simulink model "SDHDummy_IK"  (R2023b)
settings: Solver=VariableStepAuto  StartTime=0.0  StopTime=15  RelTol=1e-3
values from neighbouring files (symbols this model uses):
  m = 0.1062    [Test_New_ROBOT_dynamics.m]
  M3 = [ ... (first row only)    [ForwardPOE_Test.m]    (also in ForwardPOE_Test_2.m; Make_Mlist_2.m = M_cell{3}; Make_Slist.m = [1.00000, 0.00000, 0.00000, 0.00000; 0.00000, 0.00000, 1.000; Mlist.m = eye(4))
  T = [1 0 0 0 ... (first row only)    [DH_to_Mlist.m]    (also in ForwardKinematics.m = [T3, Gtheta * se3mat(1:3, 4) / theta; 0, 0, 0, 1]; InverseDynamics.m = [R, p; 0 0 0 1]; SDHDummy_Circle.m = transl(P(i,:)) * rpy2tr(0, 0, pi, 'xyz'); SDHDummy_Heart.m = transl(P(i,:)) * rpy2tr(0, 0, pi, 'xyz'))
  T0 = [ ... (first row only)    [SDH_Main.m]
undefined symbols (not defined in the file or in its folder): Dummy, smiData, X, Y, Z
libraries: sm_lib x594, fl_lib x22, nesl_utility x13, simulink_extras x2, robotcorelib x1
(part 11 of 11)

== system SDHDummy_IK/Subsystem/J6_STEP_1_RIGID/x35_20Motor_Assembly_1_STEP_1_RIGID/x35Motor_Driver_2_STEP_1_RIGID ==
  Dummy_0020_STEP_1_RIGID : Subsystem
  Dummy_0021_STEP_1_RIGID : Subsystem
  ReferenceFrame : sm_lib/Frames and Transforms/Reference Frame
  Transform : sm_lib/Frames and Transforms/Rigid Transform  TranslationMethod=Cartesian  TranslationStandardOffset=0  TranslationStandardOffsetUnits=m  TranslationStandardAxis=+Z  TranslationCartesianOffset=smiData.RigidTransform(111).translation  TranslationCartesianOffsetUnits=mm  TranslationROffset=0  TranslationROffsetUnits=m  TranslationZOffset=0  TranslationZOffsetUnits=m  TranslationThetaOffset=0  TranslationThetaOffsetUnits=deg  RotationMethod=ArbitraryAxis  RotationAngleUnits=rad  RotationStandardAxis=+Z  RotationAngle=smiData.RigidTransform(111).angle  RotationArbitraryAxis=smiData.RigidTransform(111).axis  FollAlignAxisA=+X  BaseAlignAxisA=+Y  FollAlignAxisB=+Y  BaseAlignAxisB=+Z  RotationSequenceAxes=FollowerAxes  RotationSequence=XYX  RotationSequenceAngles=[0 0 0]  RotationSequenceAnglesUnits=deg  RotationMatrix=[1 0 0; 0 1 0; 0 0 1]  Quaternion=[1 0 0 0]
  Transform1 : sm_lib/Frames and Transforms/Rigid Transform  TranslationMethod=Cartesian  TranslationStandardOffset=0  TranslationStandardOffsetUnits=m  TranslationStandardAxis=+Z  TranslationCartesianOffset=smiData.RigidTransform(112).translation  TranslationCartesianOffsetUnits=mm  TranslationROffset=0  TranslationROffsetUnits=m  TranslationZOffset=0  TranslationZOffsetUnits=m  TranslationThetaOffset=0  TranslationThetaOffsetUnits=deg  RotationMethod=ArbitraryAxis  RotationAngleUnits=rad  RotationStandardAxis=+Z  RotationAngle=smiData.RigidTransform(112).angle  RotationArbitraryAxis=smiData.RigidTransform(112).axis  FollAlignAxisA=+X  BaseAlignAxisA=+Y  FollAlignAxisB=+Y  BaseAlignAxisB=+Z  RotationSequenceAxes=FollowerAxes  RotationSequence=XYX  RotationSequenceAngles=[0 0 0]  RotationSequenceAnglesUnits=deg  RotationMatrix=[1 0 0; 0 1 0; 0 0 1]  Quaternion=[1 0 0 0]
  Transform2 : sm_lib/Frames and Transforms/Rigid Transform  TranslationMethod=Cartesian  TranslationStandardOffset=0  TranslationStandardOffsetUnits=m  TranslationStandardAxis=+Z  TranslationCartesianOffset=smiData.RigidTransform(113).translation  TranslationCartesianOffsetUnits=mm  TranslationROffset=0  TranslationROffsetUnits=m  TranslationZOffset=0  TranslationZOffsetUnits=m  TranslationThetaOffset=0  TranslationThetaOffsetUnits=deg  RotationMethod=ArbitraryAxis  RotationAngleUnits=rad  RotationStandardAxis=+Z  RotationAngle=smiData.RigidTransform(113).angle  RotationArbitraryAxis=smiData.RigidTransform(113).axis  FollAlignAxisA=+X  BaseAlignAxisA=+Y  FollAlignAxisB=+Y  BaseAlignAxisB=+Z  RotationSequenceAxes=FollowerAxes  RotationSequence=XYX  RotationSequenceAngles=[0 0 0]  RotationSequenceAnglesUnits=deg  RotationMatrix=[1 0 0; 0 1 0; 0 0 1]  Quaternion=[1 0 0 0]
  F : PMIOPort  Side=Left
  connections:
  Dummy_0020_STEP_1_RIGID/LConn1 -- Transform/RConn1
  Dummy_0021_STEP_1_RIGID/LConn1 -- Transform1/RConn1
  ReferenceFrame/RConn1 -- Transform/LConn1 -- Transform1/LConn1 -- Transform2/RConn1
  Transform2/LConn1 -- F/RConn1

== system SDHDummy_IK/Subsystem/J6_STEP_1_RIGID/x35_20Motor_Assembly_1_STEP_1_RIGID/x35_20_STEP_1_RIGID ==
  ReferenceFrame : sm_lib/Frames and Transforms/Reference Frame
  Solid : sm_lib/Body Elements/File Solid  ExtGeomFileName=35-20步进电机.STEP_默认_sldprt.STEP  UnitType=FromFile  ExtGeomFileUnits=m  StepReaderType=HEX  ExportConvexHullGeometry=off  InertiaType=Custom  Mass=smiData.Solid(31).mass  MassUnits=kg  CenterOfMass=smiData.Solid(31).CoM  CenterOfMassUnits=mm  MomentsOfInertia=smiData.Solid(31).MoI  MomentsOfInertiaUnits=kg*mm^2  ProductsOfInertia=smiData.Solid(31).PoI  ProductsOfInertiaUnits=kg*mm^2  BasedOnType=DensityFromFile  Density=1000  DensityUnits=kg/m^3  DoExposeReferenceFrame=on  SerializedFrames=<Frames/>  GraphicType=FromGeometry  MarkerShape=Sphere  MarkerSize=10  GraphicVisPropType=SimpleVisualProperties  GraphicDiffuseColor=smiData.Solid(31).color  GraphicSpecularColor=[0.5 0.5 0.5 1.0]  GraphicAmbientColor=[0.15 0.15 0.15 1.0]  GraphicEmissiveColor=[0.0 0.0 0.0 1.0]  GraphicShininess=75  GraphicOpacity=smiData.Solid(31).opacity
  F : PMIOPort  Side=Left
  connections:
  ReferenceFrame/RConn1 -- Solid/RConn1 -- F/RConn1

== system SDHDummy_IK/Subsystem/J4_STEP_1_RIGID/x35_28Motor_Assembly_STEP_1_RIGID/x35Motor_Driver_STEP_1_RIGID/Dummy_0020_STEP_1_RIGID ==
  ReferenceFrame : sm_lib/Frames and Transforms/Reference Frame
  Solid : sm_lib/Body Elements/File Solid  ExtGeomFileName=Dummy-0020.STEP_默认_sldprt.STEP  UnitType=FromFile  ExtGeomFileUnits=m  StepReaderType=HEX  ExportConvexHullGeometry=off  InertiaType=Custom  Mass=smiData.Solid(23).mass  MassUnits=kg  CenterOfMass=smiData.Solid(23).CoM  CenterOfMassUnits=mm  MomentsOfInertia=smiData.Solid(23).MoI  MomentsOfInertiaUnits=kg*mm^2  ProductsOfInertia=smiData.Solid(23).PoI  ProductsOfInertiaUnits=kg*mm^2  BasedOnType=DensityFromFile  Density=1000  DensityUnits=kg/m^3  DoExposeReferenceFrame=on  SerializedFrames=<Frames/>  GraphicType=FromGeometry  MarkerShape=Sphere  MarkerSize=10  GraphicVisPropType=SimpleVisualProperties  GraphicDiffuseColor=smiData.Solid(23).color  GraphicSpecularColor=[0.5 0.5 0.5 1.0]  GraphicAmbientColor=[0.15 0.15 0.15 1.0]  GraphicEmissiveColor=[0.0 0.0 0.0 1.0]  GraphicShininess=75  GraphicOpacity=smiData.Solid(23).opacity
  F : PMIOPort  Side=Left
  connections:
  ReferenceFrame/RConn1 -- Solid/RConn1 -- F/RConn1

== system SDHDummy_IK/Subsystem/J4_STEP_1_RIGID/x35_28Motor_Assembly_STEP_1_RIGID/x35Motor_Driver_STEP_1_RIGID/Dummy_0021_STEP_1_RIGID ==
  ReferenceFrame : sm_lib/Frames and Transforms/Reference Frame
  Solid : sm_lib/Body Elements/File Solid  ExtGeomFileName=Dummy-0021.STEP_默认_sldprt.STEP  UnitType=FromFile  ExtGeomFileUnits=m  StepReaderType=HEX  ExportConvexHullGeometry=off  InertiaType=Custom  Mass=smiData.Solid(24).mass  MassUnits=kg  CenterOfMass=smiData.Solid(24).CoM  CenterOfMassUnits=mm  MomentsOfInertia=smiData.Solid(24).MoI  MomentsOfInertiaUnits=kg*mm^2  ProductsOfInertia=smiData.Solid(24).PoI  ProductsOfInertiaUnits=kg*mm^2  BasedOnType=DensityFromFile  Density=1000  DensityUnits=kg/m^3  DoExposeReferenceFrame=on  SerializedFrames=<Frames/>  GraphicType=FromGeometry  MarkerShape=Sphere  MarkerSize=10  GraphicVisPropType=SimpleVisualProperties  GraphicDiffuseColor=smiData.Solid(24).color  GraphicSpecularColor=[0.5 0.5 0.5 1.0]  GraphicAmbientColor=[0.15 0.15 0.15 1.0]  GraphicEmissiveColor=[0.0 0.0 0.0 1.0]  GraphicShininess=75  GraphicOpacity=smiData.Solid(24).opacity
  F : PMIOPort  Side=Left
  connections:
  ReferenceFrame/RConn1 -- Solid/RConn1 -- F/RConn1

== system SDHDummy_IK/Subsystem/J5_STEP_1_RIGID/x35_20Motor_Assembly_STEP_1_RIGID/x35Motor_Driver_1_STEP_1_RIGID/Dummy_0020_STEP_1_RIGID ==
  ReferenceFrame : sm_lib/Frames and Transforms/Reference Frame
  Solid : sm_lib/Body Elements/File Solid  ExtGeomFileName=Dummy-0020.STEP_默认_sldprt.STEP  UnitType=FromFile  ExtGeomFileUnits=m  StepReaderType=HEX  ExportConvexHullGeometry=off  InertiaType=Custom  Mass=smiData.Solid(23).mass  MassUnits=kg  CenterOfMass=smiData.Solid(23).CoM  CenterOfMassUnits=mm  MomentsOfInertia=smiData.Solid(23).MoI  MomentsOfInertiaUnits=kg*mm^2  ProductsOfInertia=smiData.Solid(23).PoI  ProductsOfInertiaUnits=kg*mm^2  BasedOnType=DensityFromFile  Density=1000  DensityUnits=kg/m^3  DoExposeReferenceFrame=on  SerializedFrames=<Frames/>  GraphicType=FromGeometry  MarkerShape=Sphere  MarkerSize=10  GraphicVisPropType=SimpleVisualProperties  GraphicDiffuseColor=smiData.Solid(23).color  GraphicSpecularColor=[0.5 0.5 0.5 1.0]  GraphicAmbientColor=[0.15 0.15 0.15 1.0]  GraphicEmissiveColor=[0.0 0.0 0.0 1.0]  GraphicShininess=75  GraphicOpacity=smiData.Solid(23).opacity
  F : PMIOPort  Side=Left
  connections:
  ReferenceFrame/RConn1 -- Solid/RConn1 -- F/RConn1

== system SDHDummy_IK/Subsystem/J5_STEP_1_RIGID/x35_20Motor_Assembly_STEP_1_RIGID/x35Motor_Driver_1_STEP_1_RIGID/Dummy_0021_STEP_1_RIGID ==
  ReferenceFrame : sm_lib/Frames and Transforms/Reference Frame
  Solid : sm_lib/Body Elements/File Solid  ExtGeomFileName=Dummy-0021.STEP_默认_sldprt.STEP  UnitType=FromFile  ExtGeomFileUnits=m  StepReaderType=HEX  ExportConvexHullGeometry=off  InertiaType=Custom  Mass=smiData.Solid(24).mass  MassUnits=kg  CenterOfMass=smiData.Solid(24).CoM  CenterOfMassUnits=mm  MomentsOfInertia=smiData.Solid(24).MoI  MomentsOfInertiaUnits=kg*mm^2  ProductsOfInertia=smiData.Solid(24).PoI  ProductsOfInertiaUnits=kg*mm^2  BasedOnType=DensityFromFile  Density=1000  DensityUnits=kg/m^3  DoExposeReferenceFrame=on  SerializedFrames=<Frames/>  GraphicType=FromGeometry  MarkerShape=Sphere  MarkerSize=10  GraphicVisPropType=SimpleVisualProperties  GraphicDiffuseColor=smiData.Solid(24).color  GraphicSpecularColor=[0.5 0.5 0.5 1.0]  GraphicAmbientColor=[0.15 0.15 0.15 1.0]  GraphicEmissiveColor=[0.0 0.0 0.0 1.0]  GraphicShininess=75  GraphicOpacity=smiData.Solid(24).opacity
  F : PMIOPort  Side=Left
  connections:
  ReferenceFrame/RConn1 -- Solid/RConn1 -- F/RConn1

== system SDHDummy_IK/Subsystem/J6_STEP_1_RIGID/x35_20Motor_Assembly_1_STEP_1_RIGID/x35Motor_Driver_2_STEP_1_RIGID/Dummy_0020_STEP_1_RIGID ==
  ReferenceFrame : sm_lib/Frames and Transforms/Reference Frame
  Solid : sm_lib/Body Elements/File Solid  ExtGeomFileName=Dummy-0020.STEP_默认_sldprt.STEP  UnitType=FromFile  ExtGeomFileUnits=m  StepReaderType=HEX  ExportConvexHullGeometry=off  InertiaType=Custom  Mass=smiData.Solid(23).mass  MassUnits=kg  CenterOfMass=smiData.Solid(23).CoM  CenterOfMassUnits=mm  MomentsOfInertia=smiData.Solid(23).MoI  MomentsOfInertiaUnits=kg*mm^2  ProductsOfInertia=smiData.Solid(23).PoI  ProductsOfInertiaUnits=kg*mm^2  BasedOnType=DensityFromFile  Density=1000  DensityUnits=kg/m^3  DoExposeReferenceFrame=on  SerializedFrames=<Frames/>  GraphicType=FromGeometry  MarkerShape=Sphere  MarkerSize=10  GraphicVisPropType=SimpleVisualProperties  GraphicDiffuseColor=smiData.Solid(23).color  GraphicSpecularColor=[0.5 0.5 0.5 1.0]  GraphicAmbientColor=[0.15 0.15 0.15 1.0]  GraphicEmissiveColor=[0.0 0.0 0.0 1.0]  GraphicShininess=75  GraphicOpacity=smiData.Solid(23).opacity
  F : PMIOPort  Side=Left
  connections:
  ReferenceFrame/RConn1 -- Solid/RConn1 -- F/RConn1

== system SDHDummy_IK/Subsystem/J6_STEP_1_RIGID/x35_20Motor_Assembly_1_STEP_1_RIGID/x35Motor_Driver_2_STEP_1_RIGID/Dummy_0021_STEP_1_RIGID ==
  ReferenceFrame : sm_lib/Frames and Transforms/Reference Frame
  Solid : sm_lib/Body Elements/File Solid  ExtGeomFileName=Dummy-0021.STEP_默认_sldprt.STEP  UnitType=FromFile  ExtGeomFileUnits=m  StepReaderType=HEX  ExportConvexHullGeometry=off  InertiaType=Custom  Mass=smiData.Solid(24).mass  MassUnits=kg  CenterOfMass=smiData.Solid(24).CoM  CenterOfMassUnits=mm  MomentsOfInertia=smiData.Solid(24).MoI  MomentsOfInertiaUnits=kg*mm^2  ProductsOfInertia=smiData.Solid(24).PoI  ProductsOfInertiaUnits=kg*mm^2  BasedOnType=DensityFromFile  Density=1000  DensityUnits=kg/m^3  DoExposeReferenceFrame=on  SerializedFrames=<Frames/>  GraphicType=FromGeometry  MarkerShape=Sphere  MarkerSize=10  GraphicVisPropType=SimpleVisualProperties  GraphicDiffuseColor=smiData.Solid(24).color  GraphicSpecularColor=[0.5 0.5 0.5 1.0]  GraphicAmbientColor=[0.15 0.15 0.15 1.0]  GraphicEmissiveColor=[0.0 0.0 0.0 1.0]  GraphicShininess=75  GraphicOpacity=smiData.Solid(24).opacity
  F : PMIOPort  Side=Left
  connections:
  ReferenceFrame/RConn1 -- Solid/RConn1 -- F/RConn1

== matlab function SDHDummy_IK/MATLAB Function ==
  data: all_solutions input; optimal_joint output; current_joint input
function optimal_joint = ur5_select_optimal_simple(all_solutions, current_joint)
%#codegen
%UR5_SELECT_OPTIMAL_SIMPLE 从8组逆解中选择最优解（简化版）
%
%   输入:
%       all_solutions - 8x6 矩阵，8组可能的关节角解 (rad)
%       current_joint - 1x6 向量，当前关节角度 (rad)
%
%   输出:
%       optimal_joint - 1x6 向量，最优的关节角解 (rad)
%
%   选择准则:  选择与当前关节角度变化最小的有效解

    %% ================== 初始化 ==================
    NUM_SOLUTIONS = 8;
    NUM_JOINTS = 6;
    
    optimal_joint = zeros(1, NUM_JOINTS);
    min_distance = 1e10;
    best_idx = 0;

    %% ================== 遍历所有解 ==================
    for sol_idx = 1:NUM_SOLUTIONS
        
        % 检查是否为有效解（无NaN/Inf）
        is_valid = true;
        for j = 1:NUM_JOINTS
            if isnan(all_solutions(sol_idx, j)) || isinf(all_solutions(sol_idx, j))
                is_valid = false;
            end
        end
        
        if ~is_valid
            continue;
        end
        
        % 计算与当前关节角度的距离
        distance = 0;
        for j = 1:NUM_JOINTS
            % 角度差归一化
            diff = all_solutions(sol_idx, j) - current_joint(j);
            
            while diff > pi
                diff = diff - 2*pi;
            end
            while diff < -pi
                diff = diff + 2*pi;
            end
            
            distance = distance + diff^2;
        end
        distance = sqrt(distance);
        
        % 更新最优解
        if distance < min_distance
            min_distance = distance;
            best_idx = sol_idx;
        end
    end

    %% ================== 输出结果 ==================
    if best_idx > 0
        for j = 1:NUM_JOINTS
            ang = all_solutions(best_idx, j);
            while ang > pi
                ang = ang - 2*pi;
            end
            while ang < -pi
                ang = ang + 2*pi;
            end
            optimal_joint(j) = ang;
        end
    else
        % 无有效解，返回当前角度
        for j = 1:NUM_JOINTS
            optimal_joint(j) = current_joint(j);
        end
    end

end

== matlab function SDHDummy_IK/MATLAB Function2 ==
  data: q input; T_06 output
function T_06 = FKfcn(q)
% 输入 q: 关节角度向量 [theta1, theta2, theta3, theta4, theta5, theta6] (弧度)
% 输出 T_06: 末端执行器的 4x4 齐次变换矩阵

    % DH 参数定义 (根据你提供的数据)
    % theta(变量), d, a, alpha
    % 注意：q(i) 将替代 DH 表中的 theta 值
    
    %         d         a        alpha
    DH_params = [
        0.1245    0.035    -pi/2;  % Link 1
        0         0.146     0;     % Link 2
        0         0.052    -pi/2;  % Link 3
        0.117     0         pi/2;  % Link 4
        0         0        -pi/2;  % Link 5
        0.0775    0         0      % Link 6
    ];

    % 初始化变换矩阵为单位矩阵
    T_06 = eye(4);

    % 循环计算每一个连杆的变换矩阵并连乘
    % T_total = T_01 * T_12 * T_23 * T_34 * T_45 * T_56
    for i = 1:6
        theta = q(i);           % 当前关节角
        d     = DH_params(i, 1);
        a     = DH_params(i, 2);
        alpha = DH_params(i, 3);
        
        % 预计算三角函数以提高效率
        ct = cos(theta);
        st = sin(theta);
        ca = cos(alpha);
        sa = sin(alpha);
        
        % 标准 DH (Standard DH) 变换矩阵公式
        % T(i-1 -> i) = Rot_z(theta) * Trans_z(d) * Trans_x(a) * Rot_x(alpha)
        Ti = [
            ct,   -st*ca,   st*sa,   a*ct;
            st,    ct*ca,  -ct*sa,   a*st;
             0,       sa,      ca,      d;
             0,        0,       0,      1
        ];
        
        % 矩阵链乘
        T_06 = T_06 * Ti;
    end
end

== matlab function SDHDummy_IK/MATLAB Function3 ==
  data: q input; T_06 output
function T_06 = FKfcn(q)
% 输入 q: 关节角度向量 [theta1, theta2, theta3, theta4, theta5, theta6] (弧度)
% 输出 T_06: 末端执行器的 4x4 齐次变换矩阵

    % DH 参数定义 (根据你提供的数据)
    % theta(变量), d, a, alpha
    % 注意：q(i) 将替代 DH 表中的 theta 值
    
    %         d         a        alpha
    DH_params = [
        0.1245    0.035    -pi/2;  % Link 1
        0         0.146     0;     % Link 2
        0         0.052    -pi/2;  % Link 3
        0.117     0         pi/2;  % Link 4
        0         0        -pi/2;  % Link 5
        0.0775    0         0      % Link 6
    ];

    % 初始化变换矩阵为单位矩阵
    T_06 = eye(4);

    % 循环计算每一个连杆的变换矩阵并连乘
    % T_total = T_01 * T_12 * T_23 * T_34 * T_45 * T_56
    for i = 1:6
        theta = q(i);           % 当前关节角
        d     = DH_params(i, 1);
        a     = DH_params(i, 2);
        alpha = DH_params(i, 3);
        
        % 预计算三角函数以提高效率
        ct = cos(theta);
        st = sin(theta);
        ca = cos(alpha);
        sa = sin(alpha);
        
        % 标准 DH (Standard DH) 变换矩阵公式
        % T(i-1 -> i) = Rot_z(theta) * Trans_z(d) * Trans_x(a) * Rot_x(alpha)
        Ti = [
            ct,   -st*ca,   st*sa,   a*ct;
            st,    ct*ca,  -ct*sa,   a*st;
             0,       sa,      ca,      d;
             0,        0,       0,      1
        ];
        
        % 矩阵链乘
        T_06 = T_06 * Ti;
    end
end

== matlab function SDHDummy_IK/MATLAB Function1 ==
  data: T input; joint_angles output; DH_params input
function joint_angles = spherical_wrist_inverse_kinematics(T, DH_params)
%#codegen
%SPHERICAL_WRIST_INVERSE_KINEMATICS 球形腕机械臂逆运动学解析解（Simulink兼容）
%
%   输入:  
%       T         - 4x4 齐次变换矩阵，表示末端执行器位姿
%       DH_params - 6x4 DH参数矩阵 [a, d, alpha, theta_offset]
%                   或 1x6 向量 [a1, a2, a3, d1, d4, d6] (简化输入)
%
%   输出:
%       joint_angles - 8x6 矩阵，每行为一组可能的关节角解 [θ1,θ2,θ3,θ4,θ5,θ6] (rad)
%
%   适用条件: 
%       腕部三轴相交（Pieper准则）的6轴机械臂
%       
%   解的结构 (8组解):
%       θ1: 2个解 (左臂/右臂)
%       θ3: 2个解 (肘上/肘下)  
%       θ5: 2个解 (腕正/腕反)

    %% ================== 提取DH参数 ==================
    % 支持两种输入格式
    if size(DH_params, 1) == 6 && size(DH_params, 2) >= 2
        % 完整DH参数矩阵格式 [a, d, alpha, theta_offset]
        a1 = DH_params(1, 1);
        a2 = DH_params(2, 1);
        a3 = DH_params(3, 1);
        d1 = DH_params(1, 2);
        d4 = DH_params(4, 2);
        d6 = DH_params(6, 2);
    else
        % 简化向量格式 [a1, a2, a3, d1, d4, d6]
        a1 = DH_params(1);
        a2 = DH_params(2);
        a3 = DH_params(3);
        d1 = DH_params(4);
        d4 = DH_params(5);
        d6 = DH_params(6);
    end

    %% ================== 提取变换矩阵元素 ==================
    % 旋转矩阵 R = [n, o, a]
    nx = T(1,1);  ny = T(2,1);  nz = T(3,1);    % 法向量 (normal)
    ox = T(1,2);  oy = T(2,2);  oz = T(3,2);    % 方向向量 (orientation)
    ax = T(1,3);  ay = T(2,3);  az = T(3,3);    % 接近向量 (approach)
    
    % 位置向量 p
    px = T(1,4);  py = T(2,4);  pz = T(3,4);

    %% ================== 初始化变量 ==================
    joint_angles = zeros(8, 6);
    theta1_sol = zeros(1, 2);
    theta3_sol = zeros(2, 2);
    theta2_sol = zeros(2, 2);
    theta5_sol = zeros(2, 2, 2);
    theta4_sol = zeros(2, 2, 2);
    theta6_sol = zeros(2, 2, 2);

    %% ================== 计算腕心位置 ==================
    % 腕心 = 末端位置 - d6 * 接近向量
    pwx = px - d6 * ax;
    pwy = py - d6 * ay;
    pwz = pz - d6 * az;

    %% ================== 第一阶段：位置求解 ==================
    
    %% -------- 求解 θ1 --------
    % θ1 = atan2(pwy, pwx)
    % 两个解：θ1 和 θ1 + π (左臂/右臂配置)
    
    theta1_sol(1) = atan2(pwy, pwx);
    theta1_sol(2) = atan2(-pwy, -pwx);  % 等价于 θ1 + π
    
    %% -------- 求解 θ3 和 θ2 (对每个θ1) --------
    for i = 1:2
        theta1 = theta1_sol(i);
        c1 = cos(theta1);
        s1 = sin(theta1);
        
        % 计算中间变量 A 和 B
        A = c1 * pwx + s1 * pwy - a1;
        B = -pwz + d1;
        
        % 求解 θ3
        % A² + B² = a2² + a3² + d4² + 2*a2*(a3*c3 - d4*s3)
        % 令 K = (A² + B² - a2² - a3² - d4²) / (2*a2)
        % 则 a3*c3 - d4*s3 = K
        % 转换为 ρ*cos(θ3 + φ) = K，其中 ρ = √(a3² + d4²), φ = atan2(d4, a3)
        
        K_val = (A*A + B*B - a2*a2 - a3*a3 - d4*d4) / (2 * a2);
        rho = sqrt(a3*a3 + d4*d4);
        phi = atan2(d4, a3);
        
        % 检查解的存在性
        cos_arg = K_val / rho;
        
        % 限制cos参数范围
        if cos_arg > 1
            cos_arg = 1;
        elseif cos_arg < -1
            cos_arg = -1;
        end
        
        % θ3 的两个解 (肘上/肘下)
        theta3_sol(i, 1) =  acos(cos_arg) - phi;  % 肘上
        theta3_sol(i, 2) = -acos(cos_arg) - phi;  % 肘下
        
        % 对每个θ3求解θ2
        for j = 1:2
            theta3 = theta3_sol(i, j);
            c3 = cos(theta3);
            s3 = sin(theta3);
            
            % 计算 k1 和 k2
            % k1 = a2 + a3*c3 - d4*s3
            % k2 = a3*s3 + d4*c3
            k1 = a2 + a3*c3 - d4*s3;
            k2 = a3*s3 + d4*c3;
            
            % θ2 = atan2(k1*B - k2*A, k1*A + k2*B)
            sin_theta2_num = k1*B - k2*A;
            cos_theta2_num = k1*A + k2*B;
            
            theta2_sol(i, j) = atan2(sin_theta2_num, cos_theta2_num);
        end
    end

    %% ================== 第二阶段：姿态求解 ==================
    
    for i = 1:2          % θ1 索引
        for j = 1:2      % θ3 索引
            theta1 = theta1_sol(i);
            theta2 = theta2_sol(i, j);
            theta3 = theta3_sol(i, j);
            
            c1 = cos(theta1);
            s1 = sin(theta1);
            
            % 计算 θ23 = θ2 + θ3
            theta23 = theta2 + theta3;
            c23 = cos(theta23);
            s23 = sin(theta23);
            
            %% -------- 求解 θ5 --------
            % c5 = -s23*(c1*ax + s1*ay) - c23*az
            c5 = -s23*(c1*ax + s1*ay) - c23*az;
            
            % 限制cos范围
            if c5 > 1
                c5 = 1;
            elseif c5 < -1
                c5 = -1;
            end
            
            % θ5 的两个解 (腕正/腕反)
            s5_pos = sqrt(1 - c5*c5);
            theta5_sol(i, j, 1) = atan2( s5_pos, c5);  % s5 > 0
            theta5_sol(i, j, 2) = atan2(-s5_pos, c5);  % s5 < 0
            
            %% -------- 求解 θ4 和 θ6 (对每个θ5) --------
            for k = 1:2
                theta5 = theta5_sol(i, j, k);
                s5 = sin(theta5);
                
                % 检查奇异位形 (s5 ≈ 0)
                if abs(s5) < 1e-6
                    % 奇异位形：θ4 和 θ6 耦合
                    % 此时可以任意分配，通常设 θ4 = 0 或保持当前值
                    theta4_sol(i, j, k) = 0;
                    
                    % 计算 θ4 + θ6 的组合
                    % 使用 n 和 o 向量
                    s4_plus_6 = -s1*nx + c1*ny;
                    c4_plus_6 = c1*c23*nx + s1*c23*ny - s23*nz;
                    
                    if c5 > 0
                        theta6_sol(i, j, k) = atan2(s4_plus_6, c4_plus_6);
                    else
                        theta6_sol(i, j, k) = atan2(-s4_plus_6, -c4_plus_6);
                    end
                else
                    % 非奇异位形：正常求解
                    
                    % θ4 = atan2(-s1*ax + c1*ay, -c23*(c1*ax + s1*ay) + s23*az)
                    s4_s5 = -s1*ax + c1*ay;
                    c4_s5 = -c23*(c1*ax + s1*ay) + s23*az;
                    
                    theta4_sol(i, j, k) = atan2(s4_s5, c4_s5);
                    
                    % θ6 = atan2(c1*s23*ox + s1*s23*oy + c23*oz, 
                    %           -c1*s23*nx - s1*s23*ny - c23*nz)
                    s6_s5 = c1*s23*ox + s1*s23*oy + c23*oz;
                    c6_s5 = -c1*s23*nx - s1*s23*ny - c23*nz;
                    
                    theta6_sol(i, j, k) = atan2(s6_s5, c6_s5);
                end
            end
        end
    end

    %% ================== 组装8组解 ==================
    % 解的组织: 
    % 解1-2: θ1解1, θ3解1, θ5正/负
    % 解3-4: θ1解1, θ3解2, θ5正/负
    % 解5-6: θ1解2, θ3解1, θ5正/负
    % 解7-8: θ1解2, θ3解2, θ5正/负
    
    sol_idx = 1;
    for i = 1:2          % θ1 索引
        for j = 1:2      % θ3 索引
            for k = 1:2  % θ5 索引
                joint_angles(sol_idx, 1) = theta1_sol(i);
                joint_angles(sol_idx, 2) = theta2_sol(i, j);
                joint_angles(sol_idx, 3) = theta3_sol(i, j);
                joint_angles(sol_idx, 4) = theta4_sol(i, j, k);
                joint_angles(sol_idx, 5) = theta5_sol(i, j, k);
                joint_angles(sol_idx, 6) = theta6_sol(i, j, k);
                
                sol_idx = sol_idx + 1;
            end
        end
    end

    %% ================== 角度归一化 ==================
    for sol = 1:8
        for jnt = 1:6
            ang = joint_angles(sol, jnt);
            
            while ang > pi
                ang = ang - 2*pi;
            end
            while ang < -pi
                ang = ang + 2*pi;
            end
            
            joint_angles(sol, jnt) = ang;
        end
    end

end
